simulink model "combined_experiment"  (R2020a)
settings: Solver=FixedStepAuto  StartTime=0.0  StopTime=tsim  FixedStep=baseRate  RelTol=1e-3  EnableMultiTasking=on
values from neighbouring files (symbols this model uses):
  a1 = str2double(environment_file(search_start(1)+length(value)+1:search_start(1)+search_end(1)-2))    [Run_Initializer.m]
  a2 = str2double(environment_file(search_start(1)+length(value)+1:search_start(1)+search_end(1)-2))    [Run_Initializer.m]
  a3 = str2double(environment_file(search_start(1)+length(value)+1:search_start(1)+search_end(1)-2))    [Run_Initializer.m]
  b0 = str2double(environment_file(search_start(1)+length(value)+1:search_start(1)+search_end(1)-2))    [Run_Initializer.m]
  b1 = str2double(environment_file(search_start(1)+length(value)+1:search_start(1)+search_end(1)-2))    [Run_Initializer.m]
  b2 = str2double(environment_file(search_start(1)+length(value)+1:search_start(1)+search_end(1)-2))    [Run_Initializer.m]
  baseRate = 1/20    (= 0.05)    [Run_Initializer.m]
  bring_arm_to_rest_time = 3    [Run_Initializer.m]
  drop_states_BLACK = [ 2.33; 1.2; target_starting_angle]    [Run_Initializer.m]
  drop_states_BLUE = [ xLength/2+0.9; yLength/2+0.5; 0]    [Run_Initializer.m]
  drop_states_RED = [ 0.5; 1.6; pi/4]    [Run_Initializer.m]
  elbow_max_omega = shoulder_max_omega    [Run_Initializer.m]
  F_red_X_nominal = 0.2196    [Run_Initializer.m]
  F_red_Y_nominal = 0.2825    [Run_Initializer.m]
  F_thrusters_BLACK = 0.183.*ones(8,1)    [Run_Initializer.m]
  F_thrusters_BLUE = 0.183.*ones(8,1)    [Run_Initializer.m]
  F_thrusters_RED = [F_red_X_nominal; F_red_X_nominal; F_red_Y_nominal; F_red_Y_nominal; F_red_X_nominal; F_red_X_nominal; F_red_Y_nominal; F_red_Y_nominal]    [Run_Initializer.m]
  home_states_BLACK = [ 2.33; 1.2; target_starting_angle]    [Run_Initializer.m]
  home_states_BLUE = [ xLength/2-0.9; yLength/2+0.5; 0]    [Run_Initializer.m]
  home_states_RED = drop_states_RED    [Run_Initializer.m]
  I0 = str2double(environment_file(search_start(1)+length(value)+1:search_start(1)+search_end(1)-2))    [Run_Initializer.m]
  I1 = str2double(environment_file(search_start(1)+length(value)+1:search_start(1)+search_end(1)-2))    [Run_Initializer.m]
  I2 = str2double(environment_file(search_start(1)+length(value)+1:search_start(1)+search_end(1)-2))    [Run_Initializer.m]
  I3 = str2double(environment_file(search_start(1)+length(value)+1:search_start(1)+search_end(1)-2))    [Run_Initializer.m]
  init_states_BLACK = [ 2.33; 1.2; target_starting_angle]    [Run_Initializer.m]
  init_states_BLUE = [ xLength/2+0.9; yLength/2+0.5; 0]    [Run_Initializer.m]
  init_states_RED = drop_states_RED    [Run_Initializer.m]
  joint_limit_buffer_angle = 0    [Run_Initializer.m]
  Kd_tb = 0.4/5    (= 0.08)    [Run_Initializer.m]
  Kd_tblue = 0.4    [Run_Initializer.m]
  Kd_tr = 0.4    [Run_Initializer.m]
  Kd_xb = 5    [Run_Initializer.m]
  Kd_xblue = 5    [Run_Initializer.m]
  Kd_xr = 5    [Run_Initializer.m]
  Kd_yb = 5    [Run_Initializer.m]
  Kd_yblue = 5    [Run_Initializer.m]
  Kd_yr = 5    [Run_Initializer.m]
  Kp_tb = 0.1/5    (= 0.02)    [Run_Initializer.m]
  Kp_tblue = 0.1    [Run_Initializer.m]
  Kp_tr = 0.1    [Run_Initializer.m]
  Kp_xb = 2    [Run_Initializer.m]
  Kp_xblue = 2    [Run_Initializer.m]
  Kp_xr = 2    [Run_Initializer.m]
  Kp_yb = 2    [Run_Initializer.m]
  Kp_yblue = 2    [Run_Initializer.m]
  Kp_yr = 2    [Run_Initializer.m]
  m0 = str2double(environment_file(search_start(1)+length(value)+1:search_start(1)+search_end(1)-2))    [Run_Initializer.m]
  m1 = str2double(environment_file(search_start(1)+length(value)+1:search_start(1)+search_end(1)-2))    [Run_Initializer.m]
  m2 = str2double(environment_file(search_start(1)+length(value)+1:search_start(1)+search_end(1)-2))    [Run_Initializer.m]
  m3 = str2double(environment_file(search_start(1)+length(value)+1:search_start(1)+search_end(1)-2))    [Run_Initializer.m]
  max_body_omega = str2num(erase(environment_file(search_start(1)+length(value)+1:search_start(1)+search_end(1)-2),'np.'))    [Run_Initializer.m]
  max_x_velocity = str2double(environment_file(search_start(1)+length(value)+1:search_start(1)+search_end(1)-2))    [Run_Initializer.m]
  max_y_velocity = max_x_velocity    [Run_Initializer.m]
  noise_variance_BLACK = 0    [Run_Initializer.m]
  noise_variance_BLUE = 0    [Run_Initializer.m]
  noise_variance_RED = 0    [Run_Initializer.m]
  Phase0_End = Phase0_Duration    (= 5)    [Run_Initializer.m]
  Phase1_End = Phase0_Duration + Phase1_Duration    (= 10)    [Run_Initializer.m]
  Phase2_End = Phase0_Duration + Phase1_Duration +                                   Phase2_Duration    (= 25)    [Run_Initializer.m]
  Phase3_End = Phase0_Duration + Phase1_Duration +                                   Phase2_Duration + Phase3_Duration    (= 205)    [Run_Initializer.m]
  Phase3_SubPhase1_End = Phase2_End + Phase3_SubPhase1_Duration    (= 55)    [Run_Initializer.m]
  Phase3_SubPhase2_End = Phase2_End + Phase3_SubPhase1_Duration +                                   Phase3_SubPhase2_Duration    (= 85)    [Run_Initializer.m]
  Phase3_SubPhase3_End = Phase2_End + Phase3_SubPhase1_Duration +                                   Phase3_SubPhase2_Duration +                                  Phase3_SubPhase3_Duration    (= 205)    [Run_Initializer.m]
  Phase3_SubPhase4_End = Phase2_End + Phase3_SubPhase1_Duration +                                   Phase3_SubPhase2_Duration +                                  Phase3_SubPhase3_Duration +                                  Phase3_SubPhase4_Duration    [Run_Initializer.m]
  Phase4_End = Phase0_Duration + Phase1_Duration +                                   Phase2_Duration + Phase3_Duration +                                   Phase4_Duration    (= 225)    [Run_Initializer.m]
  Phase5_End = Phase0_Duration + Phase1_Duration +                                   Phase2_Duration + Phase3_Duration +                                   Phase4_Duration + Phase5_Duration    (= 230)    [Run_Initializer.m]
  phi = str2num(erase(environment_file(search_start(1)+length(value)+1:search_start(1)+search_end(1)-2),'np.'))    [Run_Initializer.m]
  serverRate = 1/10    (= 0.1)    [Run_Initializer.m]
  shoulder_max_omega = str2num(erase(environment_file(search_start(1)+length(value)+1:search_start(1)+search_end(1)-2),'np.'))    [Run_Initializer.m]
  target_angular_velocity = -5*pi/180    (= -0.0872664625997)    [Run_Initializer.m]
  thruster_dist2CG_BLACK = [72.80;-65.20;61.75;-79.75;65.20;-65.20;74.25;-54.75]    [Run_Initializer.m]
  thruster_dist2CG_BLUE = [83.42;-52.58;55.94;-60.05;54.08;-53.92;77.06;-55.94]    [Run_Initializer.m]
  thruster_dist2CG_RED = [69.38;-56.62;50.01;-81.49;61.12;-68.38;78.99;-52.01]    [Run_Initializer.m]
  wrist_max_omega = shoulder_max_omega    [Run_Initializer.m]
undefined symbols (not defined in the file or in its folder): DiscIntNeverNeededParam, KI_vel_PI, KI_vel_PI_theta, Kp_vel_PI, Kp_vel_PI_theta, platformSelection, simMode, WhoAmI
libraries: dspstat3 x18, dspsigops x12, embdlinuxlib x10, raspberrypiBasiclib x10, MainLibrary x9, simulink x8, mspfiltlib x3, dsparch4 x3, dspswit3 x2, sensehatlib x1
(part 6 of 13)

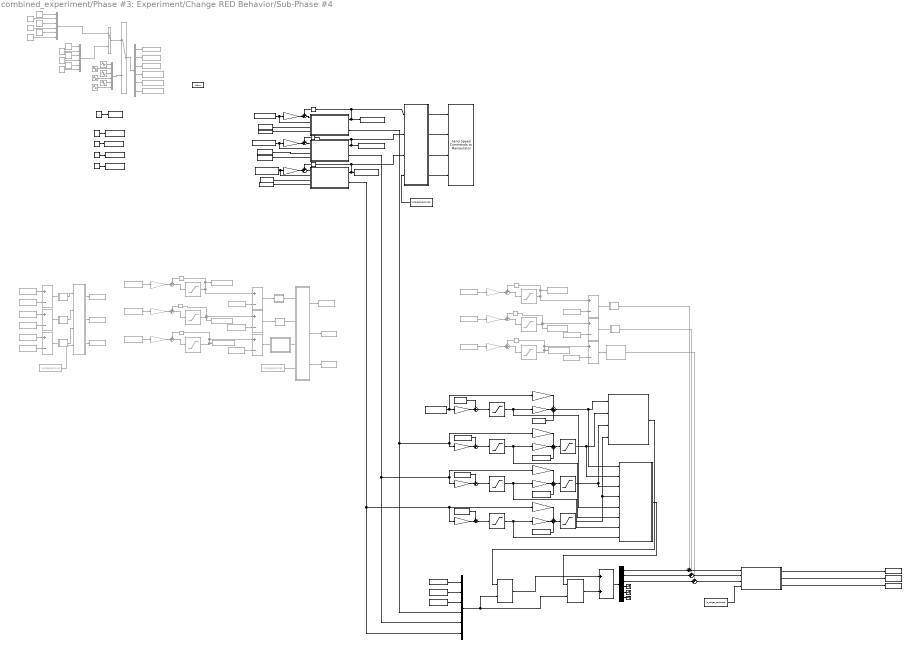
== system combined_experiment/Phase #3: Experiment/Change RED Behavior/Sub-Phase #4 ==
  note: desired q0
  note: desired q0_dot
      | (saturated)
  note: ARM Control Law - RED
  note: Acceleration-integral control law
  note: Additional Blocks
  note: Additional blocks are stored above. Note that to control attitude using the RW, simply replace RED_Tz with RED_Tz_RW.
  note: A simple PD control law is used here to command the platform to it's initial position, as defined in the initializer.
  note: This section is reserved for any control law for the robotic manipulator.
  note: Integrate and saturate acceleration signals to get desired velocities
  note: Velocity-PI control law
  note: Actually control it here
  note: Feedforward control
  note: desired q1_dot
      | (saturated)
  note: desired q1
  note: desired q2_dot
      | (saturated)
  note: desired q2
  note: desired q3_dot
      | (saturated)
  note: desired q3
  note: Velocity-PI control law
  note: Actually control it here
  note: OPTIONAL ADDITIONAL FEEDBACK VELOCITY PROPORTIONAL CONTROL
  Action Port : ActionPort  ActionPortLabel=elseif( u1 < u5)
  Check limits : MATLAB Function  TreatAsAtomicUnit=on
  Check limits1 : MATLAB Function  TreatAsAtomicUnit=on
  Check limits2 : MATLAB Function  TreatAsAtomicUnit=on
  Constant : Constant  Commented=on  Value=0.01
  Constant{1,4..6} (4 alike) : Constant  Value=0
  Constant2 : Constant  Commented=on  Value=-0.005
  Constant3 : Constant  Commented=on  Value=0.015
  Constant7 : Constant  Commented=on  Value=0.01
  Constant8 : Constant  Commented=on  Value=-0.01
  Constant9 : Constant  Commented=on  Value=0.01
  Custom Integral Acceleration Controller : Subsystem  Commented=on
  Custom Integral Acceleration Controller1 : Subsystem  Commented=on
  Custom Integral Acceleration Controller2 : Subsystem  Commented=on
  Data Store Read : DataStoreRead  DataStoreName=RED_Desired_alpha1
  Data Store Read1 : DataStoreRead  DataStoreName=RED_Desired_alpha2
  Data Store Read10 : DataStoreRead  DataStoreName=RED_omega3
  Data Store Read11 : DataStoreRead  DataStoreName=RED_omega2
  Data Store Read12 : DataStoreRead  DataStoreName=RED_omega1
  Data Store Read13 : DataStoreRead  DataStoreName=RED_theta3
  Data Store Read14 : DataStoreRead  DataStoreName=RED_theta2
  Data Store Read15 : DataStoreRead  DataStoreName=RED_theta1
  Data Store Read17 : DataStoreRead  Commented=on  DataStoreName=RED_Vx
  Data Store Read18 : DataStoreRead  Commented=on  DataStoreName=RED_Vy
  Data Store Read19 : DataStoreRead  DataStoreName=RED_theta1
  Data Store Read2 : DataStoreRead  DataStoreName=RED_Desired_alpha3
  Data Store Read20 : DataStoreRead  DataStoreName=RED_theta2
  Data Store Read21 : DataStoreRead  DataStoreName=RED_theta3
  Data Store Read22 : DataStoreRead  DataStoreName=RED_omega1
  Data Store Read23 : DataStoreRead  DataStoreName=RED_omega2
  Data Store Read24 : DataStoreRead  DataStoreName=RED_omega3
  Data Store Read25 : DataStoreRead  Commented=on  DataStoreName=RED_RzD
  Data Store Read26 : DataStoreRead  DataStoreName=RED_RzD
  Data Store Read27 : DataStoreRead  DataStoreName=RED_Rz
  Data Store Read3 : DataStoreRead  Commented=on  DataStoreName=is_target_captured
  Data Store Read4 : DataStoreRead  DataStoreName=is_target_captured
  Data Store Read5 : DataStoreRead  Commented=on  DataStoreName=is_target_captured
  Data Store Read6 : DataStoreRead  Commented=on  DataStoreName=RED_Vx
  Data Store Read7 : DataStoreRead  Commented=on  DataStoreName=RED_Vy
  Data Store Read8 : DataStoreRead  Commented=on  DataStoreName=RED_RzD
  Data Store Read9 : DataStoreRead  DataStoreName=is_target_captured
  Data Store Write : DataStoreWrite  DataStoreName=RED_Tz_Shoulder
  Data Store Write1 : DataStoreWrite  DataStoreName=RED_Tz_Elbow
  Data Store Write10 : DataStoreWrite  DataStoreName=RED_omega1_command
  Data Store Write11 : DataStoreWrite  DataStoreName=RED_omega2_command
  Data Store Write12 : DataStoreWrite  DataStoreName=RED_omega3_command
  Data Store Write13 : DataStoreWrite  Commented=on  DataStoreName=RED_Desired_Ax
  Data Store Write14 : DataStoreWrite  Commented=on  DataStoreName=RED_Desired_Ay
  Data Store Write15 : DataStoreWrite  Commented=on  DataStoreName=RED_Desired_Alpha
  Data Store Write16 : DataStoreWrite  Commented=on  DataStoreName=RED_Vy_command
  Data Store Write17 : DataStoreWrite  Commented=on  DataStoreName=RED_RzD_command
  Data Store Write18 : DataStoreWrite  Commented=on  DataStoreName=RED_Vx_command
  Data Store Write19 : DataStoreWrite  Commented=on  DataStoreName=RED_Desired_alpha1
  Data Store Write2 : DataStoreWrite  DataStoreName=RED_Tz_Wrist
  Data Store Write20 : DataStoreWrite  Commented=on  DataStoreName=RED_Desired_alpha2
  Data Store Write21 : DataStoreWrite  Commented=on  DataStoreName=RED_Desired_alpha3
  Data Store Write22 : DataStoreWrite  Commented=on  DataStoreName=RED_Vy_command
  Data Store Write23 : DataStoreWrite  Commented=on  DataStoreName=RED_RzD_command
  Data Store Write24 : DataStoreWrite  Commented=on  DataStoreName=RED_Vx_command
  Data Store Write3 : DataStoreWrite  DataStoreName=Float_State
  Delay{1..2,6..9} (6 alike) : Delay  Commented=on  DelayLength=1
  Delay3 : Delay  DelayLength=1
  Delay4 : Delay  DelayLength=1
  Delay5 : Delay  DelayLength=1
  Demux : Demux  Commented=on  Outputs=6
  Demux1 : Demux  Outputs=6
  Gain{,1..2,6,8..9,11,13..14,16..17} (11 alike) : Gain  Gain=serverRate
  Gain{7,10,12,15} (4 alike) : Gain  Gain=0.5*serverRate^2
  Gain{3..5,18..20} (6 alike) : Gain  Commented=on  Gain=serverRate
  Manual Switch : ManualSwitch  Commented=on
  Manual Switch1 : ManualSwitch  Commented=on
  Mux : Mux  Commented=on  Inputs=6
  Mux1 : Mux  Commented=on  Inputs=6
  Mux2 : Mux  Commented=on  Inputs=6
  Mux3 : Mux  Inputs=6
  PI Velocity Controller Theta : Subsystem  Commented=on
  PI Velocity Controller Theta1 : Subsystem  Commented=on
  PI Velocity Controller X : Subsystem  Commented=on
  PI Velocity Controller X1 : Subsystem  Commented=on
  PI Velocity Controller X2 : Subsystem  Commented=on
  PI Velocity Controller X3 : Subsystem  Commented=on
  Product : Product  Multiplication=Matrix(*)
  Product1 : Product  Multiplication=Matrix(*)
  Puck State : Constant
  RED_Fx1 : DataStoreWrite  Commented=on  DataStoreName=RED_Fx
  RED_Fx2 : DataStoreWrite  Commented=on  DataStoreName=RED_Fx
  RED_Fx3 : DataStoreWrite  DataStoreName=RED_Fx
  RED_Fy1 : DataStoreWrite  Commented=on  DataStoreName=RED_Fy
  RED_Fy2 : DataStoreWrite  Commented=on  DataStoreName=RED_Fy
  RED_Fy3 : DataStoreWrite  DataStoreName=RED_Fy
  RED_Py 1 : DataStoreRead  Commented=on  DataStoreName=RED_Desired_Ay
  RED_Py 10 : DataStoreRead  DataStoreName=RED_Desired_Ax
  RED_Py 2 : DataStoreRead  Commented=on  DataStoreName=RED_Desired_Ay
  RED_Py 3 : DataStoreRead  Commented=on  DataStoreName=RED_Desired_Ax
  RED_Py 4 : DataStoreRead  Commented=on  DataStoreName=RED_Desired_Ax
  RED_Py 5 : DataStoreRead  Commented=on  DataStoreName=RED_Ay
  RED_Py 6 : DataStoreRead  Commented=on  DataStoreName=RED_Desired_Ay
  RED_Py 7 : DataStoreRead  Commented=on  DataStoreName=RED_Desired_Ax
  RED_Py 8 : DataStoreRead  Commented=on  DataStoreName=RED_Ax
  RED_Py 9 : DataStoreRead  DataStoreName=RED_Desired_Ay
  RED_Rz1 : DataStoreRead  Commented=on  DataStoreName=RED_Desired_Alpha
  RED_Rz2 : DataStoreRead  Commented=on  DataStoreName=RED_Desired_Alpha
  RED_Rz3 : DataStoreRead  Commented=on  DataStoreName=RED_Desired_Alpha
  RED_Rz4 : DataStoreRead  Commented=on  DataStoreName=RED_RzDD
  RED_Rz5 : DataStoreRead  DataStoreName=RED_Desired_Alpha
  RED_Rz6 : DataStoreRead  DataStoreName=RED_Desired_Alpha
  RED_Tz1 : DataStoreWrite  Commented=on  DataStoreName=RED_Tz
  RED_Tz2 : DataStoreWrite  DataStoreName=RED_Tz
  RED_Tz3 : DataStoreWrite  Commented=on  DataStoreName=RED_Tz
  RED_Tz_RW : DataStoreWrite  DataStoreName=RED_Tz_RW
  Saturage body angular velocity command1 : Saturate  UpperLimit=shoulder_max_omega  LowerLimit=-shoulder_max_omega
  Saturage body angular velocity command2 : Saturate  UpperLimit=max_body_omega  LowerLimit=-max_body_omega
  Saturage body angular velocity command3 : Saturate  UpperLimit=elbow_max_omega  LowerLimit=-elbow_max_omega
  Saturage body angular velocity command4 : Saturate  UpperLimit=wrist_max_omega  LowerLimit=-wrist_max_omega
  Saturage body angular velocity command : Saturate  Commented=on  UpperLimit=max_body_omega  LowerLimit=-max_body_omega
  Saturage body angular velocity command1 : Saturate  Commented=on  UpperLimit=max_body_omega  LowerLimit=-max_body_omega
  Saturate velocity command X : Saturate  Commented=on  UpperLimit=max_x_velocity  LowerLimit=-max_x_velocity
  Saturate velocity command X1 : Saturate  Commented=on  UpperLimit=max_x_velocity  LowerLimit=-max_x_velocity
  Saturate velocity command Y : Saturate  Commented=on  UpperLimit=max_y_velocity  LowerLimit=-max_y_velocity
  Saturate velocity command Y1 : Saturate  Commented=on  UpperLimit=max_y_velocity  LowerLimit=-max_y_velocity
  Send Speed Commands to Manipulator : MainLibrary/Dynamixel Functions/Send Speed Commands to  Manipulator
      settings: SourceProductName=SPOT Custom Library
  Sine Wave : Sin  Commented=on  Amplitude=0.015
  Sine Wave1 : Sin  Commented=on  Amplitude=0.015  Phase=pi
  Sine Wave2 : Sin  Commented=on  Amplitude=0.04
  Sine Wave3 : Sin  Commented=on  Amplitude=0.015
  Sine Wave4 : Sin  Commented=on  Amplitude=0.015  Phase=pi
  Sine Wave5 : Sin  Commented=on  Amplitude=0.04
  Subtract{1..9} (9 alike) : Sum  Commented=on  Inputs=+-
  Sum : Sum
  Sum{1..2,6,15..17} (6 alike) : Sum  Commented=on  Inputs=++|
  Sum{3..5,8,10,12..13,18..20} (10 alike) : Sum  Inputs=++|
  Sum{7,9,11,14} (4 alike) : Sum  Inputs=+++
  Terminator : Terminator
  Terminator1 : Terminator
  Terminator2 : Terminator
  Uniform Random Number{,1,3..4} (4 alike) : UniformRandomNumber  Commented=on  Minimum=-0.015  Maximum=0.015
  Uniform Random Number2 : UniformRandomNumber  Commented=on  Minimum=-0.04  Maximum=0.04
  Uniform Random Number5 : UniformRandomNumber  Commented=on  Minimum=-0.04  Maximum=0.04
  calculate_coriolis_matrix : MATLAB Function  TreatAsAtomicUnit=on
  calculate_mass_matrix : MATLAB Function  TreatAsAtomicUnit=on
  saturate arm angle : Saturate  UpperLimit=pi/2  LowerLimit=-pi/2
  saturate arm angle1 : Saturate  UpperLimit=pi/2  LowerLimit=-pi/2
  saturate arm angle2 : Saturate  UpperLimit=pi/2  LowerLimit=-pi/2
  wind down upon capture : MATLAB Function  TreatAsAtomicUnit=on
  wind down upon_capture : MATLAB Function  Commented=on  TreatAsAtomicUnit=on
  wind down upon_capture1 : MATLAB Function  Commented=on  TreatAsAtomicUnit=on
  wind down upon_capture2 : MATLAB Function  TreatAsAtomicUnit=on
  wires:
  Constant1/1 -> RED_Tz_RW/1
  Constant6/1 -> Data Store Write2/1
  Constant4/1 -> Data Store Write/1
  Constant5/1 -> Data Store Write1/1
  Puck State/1 -> Data Store Write3/1
  Subtract6/1 -> Custom Integral Acceleration Controller1/1(ey)
  Subtract5/1 -> Custom Integral Acceleration Controller/1(ex)
  RED_Py 8/1 -> Subtract5/2
  RED_Rz4/1 -> Subtract7/2
  Subtract7/1 -> Custom Integral Acceleration Controller2/1(ez)
  RED_Py 5/1 -> Subtract6/2
  RED_Py 3/1 -> Subtract5/1
  RED_Py 1/1 -> Subtract6/1
  RED_Rz1/1 -> Subtract7/1
  Data Store Read/1 -> Check limits/2(alpha_command), Gain/1
  Check limits/1(saturated_omega) -> wind down upon capture/1(omega1_in), Delay3/1, Data Store Write10/1
  Delay3/1 -> Sum3/1
  Gain/1 -> Sum3/2
  Sum3/1 -> Check limits/1(omega_command)
  Sum4/1 -> Check limits1/1(omega_command)
  Delay4/1 -> Sum4/1
  Gain1/1 -> Sum4/2
  Check limits1/1(saturated_omega) -> Data Store Write11/1, wind down upon capture/2(omega2_in), Delay4/1
  Sum5/1 -> Check limits2/1(omega_command)
  Delay5/1 -> Sum5/1
  Gain2/1 -> Sum5/2
  Check limits2/1(saturated_omega) -> Data Store Write12/1, wind down upon capture/3(omega3_in), Delay5/1
  Data Store Read2/1 -> Check limits2/2(alpha_command), Gain2/1
  Data Store Read1/1 -> Check limits1/2(alpha_command), Gain1/1
  Data Store Read3/1 -> wind down upon_capture/4(is_target_captured)
  Custom Integral Acceleration Controller/1(Fx) -> wind down upon_capture/1(Fx_in)
  Custom Integral Acceleration Controller1/1(Fy) -> wind down upon_capture/2(Fy_in)
  Custom Integral Acceleration Controller2/1(Tz) -> wind down upon_capture/3(Tz_in)
  wind down upon capture/4(accel_time_ms) -> Send Speed Commands to Manipulator/4
  wind down upon_capture/1(Fx_out) -> RED_Fx2/1
  wind down upon_capture/2(Fy_out) -> RED_Fy2/1
  wind down upon_capture/3(Tz_out) -> RED_Tz3/1
  Sine Wave/1 -> Mux/1
  Mux/1 -> Manual Switch/2
  Constant3/1 -> Mux1/3
  Constant2/1 -> Mux1/2
  Constant/1 -> Mux1/1
  Manual Switch/1 -> Demux/1
  Demux/1 -> Data Store Write13/1
  Demux/2 -> Data Store Write14/1
  Demux/3 -> Data Store Write15/1
  Data Store Read4/1 -> wind down upon capture/4(is_target_captured)
  Subtract2/1 -> PI Velocity Controller X1/1(e_Vx)
  PI Velocity Controller X1/1(Fx) -> wind down upon_capture1/2(Fy_in)
  wind down upon_capture1/3(Tz_out) -> RED_Tz1/1
  PI Velocity Controller Theta/1(F_omega) -> wind down upon_capture1/3(Tz_in)
  Data Store Read5/1 -> wind down upon_capture1/4(is_target_captured)
  PI Velocity Controller X/1(Fx) -> wind down upon_capture1/1(Fx_in)
  wind down upon_capture1/1(Fx_out) -> RED_Fx1/1
  Subtract1/1 -> PI Velocity Controller X/1(e_Vx)
  Subtract3/1 -> PI Velocity Controller Theta/1(e_omega)
  wind down upon_capture1/2(Fy_out) -> RED_Fy1/1
  Sum2/1 -> Saturate velocity command Y/1
  Saturate velocity command Y/1 -> Data Store Write16/1, Delay2/1, Subtract2/1
  Gain4/1 -> Sum2/2
  Gain5/1 -> Sum6/2
  Sum6/1 -> Saturage body angular velocity command/1
  Delay1/1 -> Sum1/1
  RED_Py 2/1 -> Gain4/1
  Delay6/1 -> Sum6/1
  Delay2/1 -> Sum2/1
  Gain3/1 -> Sum1/2
  Saturage body angular velocity command/1 -> Subtract3/1, Delay6/1, Data Store Write17/1
  RED_Rz2/1 -> Gain5/1
  Sum1/1 -> Saturate velocity command X/1
  RED_Py 4/1 -> Gain3/1
  Saturate velocity command X/1 -> Delay1/1, Data Store Write18/1, Subtract1/1
  Data Store Read6/1 -> Subtract1/2
  Data Store Read7/1 -> Subtract2/2
  Data Store Read8/1 -> Subtract3/2
  Manual Switch1/1 -> Manual Switch/1
  Mux1/1 -> Manual Switch1/1
  Uniform Random Number/1 -> Mux2/1
  Mux2/1 -> Manual Switch1/2
  Uniform Random Number2/1 -> Mux2/3
  Uniform Random Number1/1 -> Mux2/2
  RED_Py 10/1 -> Mux3/1
  RED_Py 9/1 -> Mux3/2
  RED_Rz5/1 -> Mux3/3
  Check limits/2(saturated_alpha) -> Mux3/4, Gain8/1, Gain10/1
  Check limits1/2(saturated_alpha) -> Gain13/1, Gain12/1, Mux3/5
  Check limits2/2(saturated_alpha) -> Gain16/1, Gain15/1, Mux3/6
  Mux3/1 -> Product1/2, Product/2
  calculate_mass_matrix/1(M) -> Product/1
  calculate_coriolis_matrix/1(C) -> Product1/1
  Product1/1 -> Sum/2
  Product/1 -> Sum/1
  Sum/1 -> Demux1/1
  Data Store Read9/1 -> wind down upon_capture2/4(is_target_captured)
  Demux1/4 -> Terminator/1
  Demux1/6 -> Terminator2/1
  Demux1/5 -> Terminator1/1
  Gain11/1 -> Sum12/2
  RED_Rz6/1 -> Gain7/1, Gain11/1
  Sum12/1 -> Saturage body angular velocity command2/1
  Data Store Read26/1 -> Sum12/1
  Saturage body angular velocity command2/1 -> calculate_coriolis_matrix/5(q0_dot_d), Gain6/1
  Gain6/1 -> Sum7/2
  Gain7/1 -> Sum7/1
  Data Store Read27/1 -> Sum7/3
  Sum7/1 -> calculate_coriolis_matrix/1(q0_d), calculate_mass_matrix/1(q0_d)
  Data Store Read22/1 -> Sum8/1
  Sum8/1 -> Saturage body angular velocity command1/1
  Gain8/1 -> Sum8/2
  Gain10/1 -> Sum9/1
  Sum9/1 -> saturate arm angle/1
  Data Store Read19/1 -> Sum9/3
  Gain9/1 -> Sum9/2
  Saturage body angular velocity command1/1 -> calculate_coriolis_matrix/6(q1_dot_d), Gain9/1
  Data Store Read20/1 -> Sum11/3
  Gain13/1 -> Sum10/2
  Sum10/1 -> Saturage body angular velocity command3/1
  Saturage body angular velocity command3/1 -> calculate_coriolis_matrix/7(q2_dot_d), Gain14/1
  Sum11/1 -> saturate arm angle1/1
  Data Store Read23/1 -> Sum10/1
  Gain14/1 -> Sum11/2
  Gain12/1 -> Sum11/1
  Data Store Read21/1 -> Sum14/3
  Gain16/1 -> Sum13/2
  Sum13/1 -> Saturage body angular velocity command4/1
  Saturage body angular velocity command4/1 -> calculate_coriolis_matrix/8(q3_dot_d), Gain17/1
  Sum14/1 -> saturate arm angle2/1
  Data Store Read24/1 -> Sum13/1
  Gain17/1 -> Sum14/2
  Gain15/1 -> Sum14/1
  saturate arm angle/1 -> calculate_mass_matrix/2(q1_d), calculate_coriolis_matrix/2(q1_d)
  saturate arm angle1/1 -> calculate_coriolis_matrix/3(q2_d), calculate_mass_matrix/3(q2_d)
  saturate arm angle2/1 -> calculate_mass_matrix/4(q3_d), calculate_coriolis_matrix/4(q3_d)
  Demux/4 -> Data Store Write19/1
  Demux/5 -> Data Store Write20/1
  Demux/6 -> Data Store Write21/1
  Constant8/1 -> Mux1/5
  Constant7/1 -> Mux1/4
  Constant9/1 -> Mux1/6
  Sine Wave1/1 -> Mux/2
  Sine Wave2/1 -> Mux/3
  Uniform Random Number4/1 -> Mux2/5
  Uniform Random Number3/1 -> Mux2/4
  Uniform Random Number5/1 -> Mux2/6
  Sine Wave4/1 -> Mux/5
  Sine Wave3/1 -> Mux/4
  Sine Wave5/1 -> Mux/6
  Delay8/1 -> Sum16/1
  Delay7/1 -> Sum15/1
  Delay9/1 -> Sum17/1
  Sum15/1 -> Saturate velocity command X1/1
  RED_Py 7/1 -> Gain18/1
  RED_Py 6/1 -> Gain19/1
  Gain18/1 -> Sum15/2
  Saturate velocity command X1/1 -> Delay7/1, Data Store Write24/1, Subtract4/1
  Gain20/1 -> Sum17/2
  Gain19/1 -> Sum16/2
  Saturate velocity command Y1/1 -> Data Store Write22/1, Delay8/1, Subtract8/1
  RED_Rz3/1 -> Gain20/1
  Sum16/1 -> Saturate velocity command Y1/1
  Saturage body angular velocity command1/1 -> Subtract9/1, Delay9/1, Data Store Write23/1
  Subtract9/1 -> PI Velocity Controller Theta1/1(e_omega)
  Subtract4/1 -> PI Velocity Controller X2/1(e_Vx)
  Data Store Read17/1 -> Subtract4/2
  PI Velocity Controller X3/1(Fx) -> Sum19/1
  Data Store Read25/1 -> Subtract9/2
  Subtract8/1 -> PI Velocity Controller X3/1(e_Vx)
  PI Velocity Controller X2/1(Fx) -> Sum18/1
  Sum17/1 -> Saturage body angular velocity command1/1
  PI Velocity Controller Theta1/1(F_omega) -> Sum20/1
  Data Store Read18/1 -> Subtract8/2
  Demux1/1 -> Sum18/2
  Sum18/1 -> wind down upon_capture2/1(Fx_in)
  Sum20/1 -> wind down upon_capture2/3(Tz_in)
  Demux1/3 -> Sum20/2
  Sum19/1 -> wind down upon_capture2/2(Fy_in)
  Demux1/2 -> Sum19/2
  wind down upon capture/2(omega2_out) -> Send Speed Commands to Manipulator/2
  wind down upon capture/1(omega1_out) -> Send Speed Commands to Manipulator/1
  wind down upon capture/3(omega3_out) -> Send Speed Commands to Manipulator/3
  Data Store Read12/1 -> Check limits/4(current_omega)
  Data Store Read15/1 -> Check limits/3(current_theta)
  Data Store Read14/1 -> Check limits1/3(current_theta)
  Data Store Read11/1 -> Check limits1/4(current_omega)
  Data Store Read13/1 -> Check limits2/3(current_theta)
  Data Store Read10/1 -> Check limits2/4(current_omega)
  wind down upon_capture2/1(Fx_out) -> RED_Fx3/1
  wind down upon_capture2/2(Fy_out) -> RED_Fy3/1
  wind down upon_capture2/3(Tz_out) -> RED_Tz2/1

== system combined_experiment/Phase #3: Experiment/Change RED Behavior/Subsystem ==
  Universal_Time : DataStoreRead  DataStoreName=Univ_Time
  Time : Outport  VectorParamsAs1DForOutWhenUnconnected=off
  wires:
  Universal_Time/1 -> Time/1

== system combined_experiment/Phase #4: Return Home/Change BLACK Behavior/Custom Discrete PD (Attitude) ==
  ez : Inport
  Sum3 : Sum
  kd_tb : Gain  Gain=Kd_tb
  kp_tb : Gain  Gain=Kp_tb
  "x_dot -> x1" : Subsystem
  Tz : Outport  VectorParamsAs1DForOutWhenUnconnected=off
  wires:
  kd_tb/1 -> Sum3/1
  Sum3/1 -> Tz/1
  kp_tb/1 -> Sum3/2
  "x_dot -> x1"/1(dy(t)/dt) -> kd_tb/1
  ez/1 -> "x_dot -> x1"/1(y(t)), kp_tb/1

== system combined_experiment/Phase #4: Return Home/Change BLACK Behavior/Custom Discrete PD (X-Position) ==
  ex : Inport
  Sum3 : Sum
  kd_xb : Gain  Gain=Kd_xb
  kp_xb : Gain  Gain=Kp_xb
  "x_dot -> x1" : Subsystem
  Fx : Outport  VectorParamsAs1DForOutWhenUnconnected=off
  wires:
  kd_xb/1 -> Sum3/1
  ex/1 -> "x_dot -> x1"/1(y(t)), kp_xb/1
  kp_xb/1 -> Sum3/2
  "x_dot -> x1"/1(dy(t)/dt) -> kd_xb/1
  Sum3/1 -> Fx/1

== system combined_experiment/Phase #4: Return Home/Change BLACK Behavior/Custom Discrete PD (Y-Position) ==
  ey : Inport
  Sum3 : Sum
  kd_yb : Gain  Gain=Kd_yb
  kp_yb : Gain  Gain=Kp_yb
  "x_dot -> x1" : Subsystem
  Fy : Outport  VectorParamsAs1DForOutWhenUnconnected=off
  wires:
  kd_yb/1 -> Sum3/1
  Sum3/1 -> Fy/1
  kp_yb/1 -> Sum3/2
  "x_dot -> x1"/1(dy(t)/dt) -> kd_yb/1
  ey/1 -> "x_dot -> x1"/1(y(t)), kp_yb/1

== system combined_experiment/Phase #4: Return Home/Change BLACK Behavior/Hough Control ==
  Ref : Inport
  Act : Inport  Port=2
  MATLAB Function2 : MATLAB Function  TreatAsAtomicUnit=on
  MATLAB Function3 : MATLAB Function  TreatAsAtomicUnit=on
  MATLAB Function4 : MATLAB Function  TreatAsAtomicUnit=on
  Subtract2 : Sum  Inputs=+-
  Err : Outport  VectorParamsAs1DForOutWhenUnconnected=off
  wires:
  MATLAB Function4/1(e_out) -> Err/1
  MATLAB Function2/1(Oy) -> MATLAB Function4/1(Oy)
  Subtract2/1 -> MATLAB Function4/2(e_in)
  MATLAB Function2/2(Ox) -> Subtract2/1
  Act/1 -> MATLAB Function3/1(z)
  Ref/1 -> MATLAB Function2/1(z)
  MATLAB Function3/1(Ox) -> Subtract2/2

== system combined_experiment/Phase #4: Return Home/Change BLUE Behavior/Custom Discrete PD (Attitude) ==
  ez : Inport
  Sum3 : Sum
  kd_tb : Gain  Gain=Kd_tblue
  kp_tb : Gain  Gain=Kp_tblue
  "x_dot -> x1" : Subsystem
  Tz : Outport  VectorParamsAs1DForOutWhenUnconnected=off
  wires:
  kd_tb/1 -> Sum3/1
  Sum3/1 -> Tz/1
  kp_tb/1 -> Sum3/2
  "x_dot -> x1"/1(dy(t)/dt) -> kd_tb/1
  ez/1 -> "x_dot -> x1"/1(y(t)), kp_tb/1

== system combined_experiment/Phase #4: Return Home/Change BLUE Behavior/Custom Discrete PD (X-Position) ==
  ex : Inport
  Sum3 : Sum
  kd_xb : Gain  Gain=Kd_xblue
  kp_xb : Gain  Gain=Kp_xblue
  "x_dot -> x1" : Subsystem
  Fx : Outport  VectorParamsAs1DForOutWhenUnconnected=off
  wires:
  kd_xb/1 -> Sum3/1
  ex/1 -> "x_dot -> x1"/1(y(t)), kp_xb/1
  kp_xb/1 -> Sum3/2
  "x_dot -> x1"/1(dy(t)/dt) -> kd_xb/1
  Sum3/1 -> Fx/1

== system combined_experiment/Phase #4: Return Home/Change BLUE Behavior/Custom Discrete PD (Y-Position) ==
  ey : Inport
  Sum3 : Sum
  kd_yb : Gain  Gain=Kd_yblue
  kp_yb : Gain  Gain=Kp_yblue
  "x_dot -> x1" : Subsystem
  Fy : Outport  VectorParamsAs1DForOutWhenUnconnected=off
  wires:
  kd_yb/1 -> Sum3/1
  Sum3/1 -> Fy/1
  kp_yb/1 -> Sum3/2
  "x_dot -> x1"/1(dy(t)/dt) -> kd_yb/1
  ey/1 -> "x_dot -> x1"/1(y(t)), kp_yb/1

== system combined_experiment/Phase #4: Return Home/Change BLUE Behavior/Hough Control ==
  Ref : Inport
  Act : Inport  Port=2
  MATLAB Function2 : MATLAB Function  TreatAsAtomicUnit=on
  MATLAB Function3 : MATLAB Function  TreatAsAtomicUnit=on
  MATLAB Function4 : MATLAB Function  TreatAsAtomicUnit=on
  Subtract2 : Sum  Inputs=+-
  Err : Outport  VectorParamsAs1DForOutWhenUnconnected=off
  wires:
  MATLAB Function4/1(e_out) -> Err/1
  MATLAB Function2/1(Oy) -> MATLAB Function4/1(Oy)
  Subtract2/1 -> MATLAB Function4/2(e_in)
  MATLAB Function2/2(Ox) -> Subtract2/1
  Act/1 -> MATLAB Function3/1(z)
  Ref/1 -> MATLAB Function2/1(z)
  MATLAB Function3/1(Ox) -> Subtract2/2

== system combined_experiment/Phase #4: Return Home/Change RED Behavior/Custom Discrete PD (Attitude) ==
  ez : Inport
  Sum3 : Sum
  kd_tr : Gain  Gain=Kd_tr
  kp_tr : Gain  Gain=Kp_tr
  "x_dot -> x1" : Subsystem
  Tz : Outport  VectorParamsAs1DForOutWhenUnconnected=off
  wires:
  kd_tr/1 -> Sum3/1
  Sum3/1 -> Tz/1
  kp_tr/1 -> Sum3/2
  "x_dot -> x1"/1(dy(t)/dt) -> kd_tr/1
  ez/1 -> "x_dot -> x1"/1(y(t)), kp_tr/1

== system combined_experiment/Phase #4: Return Home/Change RED Behavior/Custom Discrete PD (X-Position) ==
  ex : Inport
  Sum3 : Sum
  kd_xr : Gain  Gain=Kd_xr
  kp_xr : Gain  Gain=Kp_xr
  "x_dot -> x1" : Subsystem
  Fx : Outport  VectorParamsAs1DForOutWhenUnconnected=off
  wires:
  kd_xr/1 -> Sum3/1
  ex/1 -> "x_dot -> x1"/1(y(t)), kp_xr/1
  kp_xr/1 -> Sum3/2
  "x_dot -> x1"/1(dy(t)/dt) -> kd_xr/1
  Sum3/1 -> Fx/1

== system combined_experiment/Phase #4: Return Home/Change RED Behavior/Custom Discrete PD (Y-Position) ==
  ey : Inport
  Sum3 : Sum
  kd_yr : Gain  Gain=Kd_yr
  kp_yr : Gain  Gain=Kp_yr
  "x_dot -> x1" : Subsystem
  Fy : Outport  VectorParamsAs1DForOutWhenUnconnected=off
  wires:
  kd_yr/1 -> Sum3/1
  Sum3/1 -> Fy/1
  kp_yr/1 -> Sum3/2
  "x_dot -> x1"/1(dy(t)/dt) -> kd_yr/1
  ey/1 -> "x_dot -> x1"/1(y(t)), kp_yr/1

== system combined_experiment/Phase #4: Return Home/Change RED Behavior/Hough Control ==
  Ref : Inport
  Act : Inport  Port=2
  MATLAB Function2 : MATLAB Function  TreatAsAtomicUnit=on
  MATLAB Function3 : MATLAB Function  TreatAsAtomicUnit=on
  MATLAB Function4 : MATLAB Function  TreatAsAtomicUnit=on
  Subtract2 : Sum  Inputs=+-
  Err : Outport  VectorParamsAs1DForOutWhenUnconnected=off
  wires:
  MATLAB Function4/1(e_out) -> Err/1
  MATLAB Function2/1(Oy) -> MATLAB Function4/1(Oy)
  Subtract2/1 -> MATLAB Function4/2(e_in)
  MATLAB Function2/2(Ox) -> Subtract2/1
  Act/1 -> MATLAB Function3/1(z)
  Ref/1 -> MATLAB Function2/1(z)
  MATLAB Function3/1(Ox) -> Subtract2/2

== system combined_experiment/Phase #5: Hold Home/Change BLACK Behavior/Custom Discrete PD (Attitude) ==
  ez : Inport
  Sum3 : Sum
  kd_tb : Gain  Gain=Kd_tb
  kp_tb : Gain  Gain=Kp_tb
  "x_dot -> x1" : Subsystem
  Tz : Outport  VectorParamsAs1DForOutWhenUnconnected=off
  wires:
  kd_tb/1 -> Sum3/1
  Sum3/1 -> Tz/1
  kp_tb/1 -> Sum3/2
  "x_dot -> x1"/1(dy(t)/dt) -> kd_tb/1
  ez/1 -> "x_dot -> x1"/1(y(t)), kp_tb/1

== system combined_experiment/Phase #5: Hold Home/Change BLACK Behavior/Custom Discrete PD (X-Position) ==
  ex : Inport
  Sum3 : Sum
  kd_xb : Gain  Gain=Kd_xb
  kp_xb : Gain  Gain=Kp_xb
  "x_dot -> x1" : Subsystem
  Fx : Outport  VectorParamsAs1DForOutWhenUnconnected=off
  wires:
  kd_xb/1 -> Sum3/1
  ex/1 -> "x_dot -> x1"/1(y(t)), kp_xb/1
  kp_xb/1 -> Sum3/2
  "x_dot -> x1"/1(dy(t)/dt) -> kd_xb/1
  Sum3/1 -> Fx/1

== system combined_experiment/Phase #5: Hold Home/Change BLACK Behavior/Custom Discrete PD (Y-Position) ==
  ey : Inport
  Sum3 : Sum
  kd_yb : Gain  Gain=Kd_yb
  kp_yb : Gain  Gain=Kp_yb
  "x_dot -> x1" : Subsystem
  Fy : Outport  VectorParamsAs1DForOutWhenUnconnected=off
  wires:
  kd_yb/1 -> Sum3/1
  Sum3/1 -> Fy/1
  kp_yb/1 -> Sum3/2
  "x_dot -> x1"/1(dy(t)/dt) -> kd_yb/1
  ey/1 -> "x_dot -> x1"/1(y(t)), kp_yb/1

== system combined_experiment/Phase #5: Hold Home/Change BLACK Behavior/Hough Control ==
  Ref : Inport
  Act : Inport  Port=2
  MATLAB Function2 : MATLAB Function  TreatAsAtomicUnit=on
  MATLAB Function3 : MATLAB Function  TreatAsAtomicUnit=on
  MATLAB Function4 : MATLAB Function  TreatAsAtomicUnit=on
  Subtract2 : Sum  Inputs=+-
  Err : Outport  VectorParamsAs1DForOutWhenUnconnected=off
  wires:
  MATLAB Function4/1(e_out) -> Err/1
  MATLAB Function2/1(Oy) -> MATLAB Function4/1(Oy)
  Subtract2/1 -> MATLAB Function4/2(e_in)
  MATLAB Function2/2(Ox) -> Subtract2/1
  Act/1 -> MATLAB Function3/1(z)
  Ref/1 -> MATLAB Function2/1(z)
  MATLAB Function3/1(Ox) -> Subtract2/2

== system combined_experiment/Phase #5: Hold Home/Change BLUE Behavior/Custom Discrete PD (Attitude) ==
  ez : Inport
  Sum3 : Sum
  kd_tb : Gain  Gain=Kd_tblue
  kp_tb : Gain  Gain=Kp_tblue
  "x_dot -> x1" : Subsystem
  Tz : Outport  VectorParamsAs1DForOutWhenUnconnected=off
  wires:
  kd_tb/1 -> Sum3/1
  Sum3/1 -> Tz/1
  kp_tb/1 -> Sum3/2
  "x_dot -> x1"/1(dy(t)/dt) -> kd_tb/1
  ez/1 -> "x_dot -> x1"/1(y(t)), kp_tb/1

== system combined_experiment/Phase #5: Hold Home/Change BLUE Behavior/Custom Discrete PD (X-Position) ==
  ex : Inport
  Sum3 : Sum
  kd_xb : Gain  Gain=Kd_xblue
  kp_xb : Gain  Gain=Kp_xblue
  "x_dot -> x1" : Subsystem
  Fx : Outport  VectorParamsAs1DForOutWhenUnconnected=off
  wires:
  kd_xb/1 -> Sum3/1
  ex/1 -> "x_dot -> x1"/1(y(t)), kp_xb/1
  kp_xb/1 -> Sum3/2
  "x_dot -> x1"/1(dy(t)/dt) -> kd_xb/1
  Sum3/1 -> Fx/1

== system combined_experiment/Phase #5: Hold Home/Change BLUE Behavior/Custom Discrete PD (Y-Position) ==
  ey : Inport
  Sum3 : Sum
  kd_yb : Gain  Gain=Kd_yblue
  kp_yb : Gain  Gain=Kp_yblue
  "x_dot -> x1" : Subsystem
  Fy : Outport  VectorParamsAs1DForOutWhenUnconnected=off
  wires:
  kd_yb/1 -> Sum3/1
  Sum3/1 -> Fy/1
  kp_yb/1 -> Sum3/2
  "x_dot -> x1"/1(dy(t)/dt) -> kd_yb/1
  ey/1 -> "x_dot -> x1"/1(y(t)), kp_yb/1

== system combined_experiment/Phase #5: Hold Home/Change BLUE Behavior/Hough Control ==
  Ref : Inport
  Act : Inport  Port=2
  MATLAB Function2 : MATLAB Function  TreatAsAtomicUnit=on
  MATLAB Function3 : MATLAB Function  TreatAsAtomicUnit=on
  MATLAB Function4 : MATLAB Function  TreatAsAtomicUnit=on
  Subtract2 : Sum  Inputs=+-
  Err : Outport  VectorParamsAs1DForOutWhenUnconnected=off
  wires:
  MATLAB Function4/1(e_out) -> Err/1
  MATLAB Function2/1(Oy) -> MATLAB Function4/1(Oy)
  Subtract2/1 -> MATLAB Function4/2(e_in)
  MATLAB Function2/2(Ox) -> Subtract2/1
  Act/1 -> MATLAB Function3/1(z)
  Ref/1 -> MATLAB Function2/1(z)
  MATLAB Function3/1(Ox) -> Subtract2/2

== system combined_experiment/Phase #5: Hold Home/Change RED Behavior/Custom Discrete PD (Attitude) ==
  ez : Inport
  Sum3 : Sum
  kd_tr : Gain  Gain=Kd_tr
  kp_tr : Gain  Gain=Kp_tr
  "x_dot -> x1" : Subsystem
  Tz : Outport  VectorParamsAs1DForOutWhenUnconnected=off
  wires:
  kd_tr/1 -> Sum3/1
  Sum3/1 -> Tz/1
  kp_tr/1 -> Sum3/2
  "x_dot -> x1"/1(dy(t)/dt) -> kd_tr/1
  ez/1 -> "x_dot -> x1"/1(y(t)), kp_tr/1

== system combined_experiment/Phase #5: Hold Home/Change RED Behavior/Custom Discrete PD (X-Position) ==
  ex : Inport
  Sum3 : Sum
  kd_xr : Gain  Gain=Kd_xr
  kp_xr : Gain  Gain=Kp_xr
  "x_dot -> x1" : Subsystem
  Fx : Outport  VectorParamsAs1DForOutWhenUnconnected=off
  wires:
  kd_xr/1 -> Sum3/1
  ex/1 -> "x_dot -> x1"/1(y(t)), kp_xr/1
  kp_xr/1 -> Sum3/2
  "x_dot -> x1"/1(dy(t)/dt) -> kd_xr/1
  Sum3/1 -> Fx/1

== system combined_experiment/Phase #5: Hold Home/Change RED Behavior/Custom Discrete PD (Y-Position) ==
  ey : Inport
  Sum3 : Sum
  kd_yr : Gain  Gain=Kd_yr
  kp_yr : Gain  Gain=Kp_yr
  "x_dot -> x1" : Subsystem
  Fy : Outport  VectorParamsAs1DForOutWhenUnconnected=off
  wires:
  kd_yr/1 -> Sum3/1
  Sum3/1 -> Fy/1
  kp_yr/1 -> Sum3/2
  "x_dot -> x1"/1(dy(t)/dt) -> kd_yr/1
  ey/1 -> "x_dot -> x1"/1(y(t)), kp_yr/1

== system combined_experiment/Phase #5: Hold Home/Change RED Behavior/Hough Control ==
  Ref : Inport
  Act : Inport  Port=2
  MATLAB Function2 : MATLAB Function  TreatAsAtomicUnit=on
  MATLAB Function3 : MATLAB Function  TreatAsAtomicUnit=on
  MATLAB Function4 : MATLAB Function  TreatAsAtomicUnit=on
  Subtract2 : Sum  Inputs=+-
  Err : Outport  VectorParamsAs1DForOutWhenUnconnected=off
  wires:
  MATLAB Function4/1(e_out) -> Err/1
  MATLAB Function2/1(Oy) -> MATLAB Function4/1(Oy)
  Subtract2/1 -> MATLAB Function4/2(e_in)
  MATLAB Function2/2(Ox) -> Subtract2/1
  Act/1 -> MATLAB Function3/1(z)
  Ref/1 -> MATLAB Function2/1(z)
  MATLAB Function3/1(Ox) -> Subtract2/2

== system combined_experiment/Simulate Plant Dynamics/x_dot -> x1/Hold this value ==
  In1 : Inport
  Action Port : ActionPort  ActionPortLabel=if(u1 ~= 0)
  Out1 : Outport  VectorParamsAs1DForOutWhenUnconnected=off
  wires:
  In1/1 -> Out1/1

== system combined_experiment/Simulate Plant Dynamics/x_dot -> x10/Hold this value ==
  In1 : Inport
  Action Port : ActionPort  ActionPortLabel=if(u1 ~= 0)
  Out1 : Outport  VectorParamsAs1DForOutWhenUnconnected=off
  wires:
  In1/1 -> Out1/1

== system combined_experiment/Simulate Plant Dynamics/x_dot -> x11/Hold this value ==
  In1 : Inport
  Action Port : ActionPort  ActionPortLabel=if(u1 ~= 0)
  Out1 : Outport  VectorParamsAs1DForOutWhenUnconnected=off
  wires:
  In1/1 -> Out1/1

== system combined_experiment/Simulate Plant Dynamics/x_dot -> x12/Hold this value ==
  In1 : Inport
  Action Port : ActionPort  ActionPortLabel=if(u1 ~= 0)
  Out1 : Outport  VectorParamsAs1DForOutWhenUnconnected=off
  wires:
  In1/1 -> Out1/1

== system combined_experiment/Simulate Plant Dynamics/x_dot -> x13/Hold this value ==
  In1 : Inport
  Action Port : ActionPort  ActionPortLabel=if(u1 ~= 0)
  Out1 : Outport  VectorParamsAs1DForOutWhenUnconnected=off
  wires:
  In1/1 -> Out1/1

== system combined_experiment/Simulate Plant Dynamics/x_dot -> x14/Hold this value ==
  In1 : Inport
  Action Port : ActionPort  ActionPortLabel=if(u1 ~= 0)
  Out1 : Outport  VectorParamsAs1DForOutWhenUnconnected=off
  wires:
  In1/1 -> Out1/1

== system combined_experiment/Simulate Plant Dynamics/x_dot -> x16/Hold this value ==
  In1 : Inport
  Action Port : ActionPort  ActionPortLabel=if(u1 ~= 0)
  Out1 : Outport  VectorParamsAs1DForOutWhenUnconnected=off
  wires:
  In1/1 -> Out1/1

== system combined_experiment/Simulate Plant Dynamics/x_dot -> x17/Hold this value ==
  In1 : Inport
  Action Port : ActionPort  ActionPortLabel=if(u1 ~= 0)
  Out1 : Outport  VectorParamsAs1DForOutWhenUnconnected=off
  wires:
  In1/1 -> Out1/1

== system combined_experiment/Simulate Plant Dynamics/x_dot -> x2/Hold this value ==
  In1 : Inport
  Action Port : ActionPort  ActionPortLabel=if(u1 ~= 0)
  Out1 : Outport  VectorParamsAs1DForOutWhenUnconnected=off
  wires:
  In1/1 -> Out1/1

== system combined_experiment/Simulate Plant Dynamics/x_dot -> x3/Hold this value ==
  In1 : Inport
  Action Port : ActionPort  ActionPortLabel=if(u1 ~= 0)
  Out1 : Outport  VectorParamsAs1DForOutWhenUnconnected=off
  wires:
  In1/1 -> Out1/1

== system combined_experiment/Simulate Plant Dynamics/x_dot -> x4/Hold this value ==
  In1 : Inport
  Action Port : ActionPort  ActionPortLabel=if(u1 ~= 0)
  Out1 : Outport  VectorParamsAs1DForOutWhenUnconnected=off
  wires:
  In1/1 -> Out1/1

== system combined_experiment/Simulate Plant Dynamics/x_dot -> x5/Hold this value ==
  In1 : Inport
  Action Port : ActionPort  ActionPortLabel=if(u1 ~= 0)
  Out1 : Outport  VectorParamsAs1DForOutWhenUnconnected=off
  wires:
  In1/1 -> Out1/1

== system combined_experiment/Simulate Plant Dynamics/x_dot -> x6/Hold this value ==
  In1 : Inport
  Action Port : ActionPort  ActionPortLabel=if(u1 ~= 0)
  Out1 : Outport  VectorParamsAs1DForOutWhenUnconnected=off
  wires:
  In1/1 -> Out1/1

== system combined_experiment/Simulate Plant Dynamics/x_dot -> x7/Hold this value ==
  In1 : Inport
  Action Port : ActionPort  ActionPortLabel=if(u1 ~= 0)
  Out1 : Outport  VectorParamsAs1DForOutWhenUnconnected=off
  wires:
  In1/1 -> Out1/1

== system combined_experiment/Simulate Plant Dynamics/x_dot -> x8/Hold this value ==
  In1 : Inport
  Action Port : ActionPort  ActionPortLabel=if(u1 ~= 0)
  Out1 : Outport  VectorParamsAs1DForOutWhenUnconnected=off
  wires:
  In1/1 -> Out1/1

== system combined_experiment/Simulate Plant Dynamics/x_dot -> x9/Hold this value ==
  In1 : Inport
  Action Port : ActionPort  ActionPortLabel=if(u1 ~= 0)
  Out1 : Outport  VectorParamsAs1DForOutWhenUnconnected=off
  wires:
  In1/1 -> Out1/1

== system combined_experiment/From Force//Torque to PWM Signal/Change BLACK Behavior/Calculate Thruster ON//OFF/Rotate Forces to Inertial ==
  "F_b " : Inport
  Rz : Inport  Port=2
  Create Rotation Matrix : MATLAB Function  TreatAsAtomicUnit=on
  Rotate F_b to F_I : Product  Multiplication=Matrix(*)
  F_I : Outport  VectorParamsAs1DForOutWhenUnconnected=off
  wires:
  "F_b "/1 -> Rotate F_b to F_I/2
  Rotate F_b to F_I/1 -> F_I/1
  Create Rotation Matrix/1(C_Ib) -> Rotate F_b to F_I/1
  Rz/1 -> Create Rotation Matrix/1(Rz)

== system combined_experiment/From Force//Torque to PWM Signal/Change BLACK Behavior/Calculate Thruster ON//OFF/pseudo-inverse ==
  H : Inport
  Product : Product  Multiplication=Matrix(*)
  Product1 : Product  Inputs=/  Multiplication=Matrix(*)
  Product2 : Product  Multiplication=Matrix(*)
  transpose : PermuteDimensions
  invH : Outport  VectorParamsAs1DForOutWhenUnconnected=off
  wires:
  Product2/1 -> invH/1
  transpose/1 -> Product/2, Product2/1
  Product/1 -> Product1/1
  H/1 -> Product/1, transpose/1
  Product1/1 -> Product2/2

== system combined_experiment/From Force//Torque to PWM Signal/Change BLUE Behavior/Calculate Thruster ON//OFF/Rotate Forces to Inertial ==
  "F_b " : Inport
  Rz : Inport  Port=2
  Create Rotation Matrix : MATLAB Function  TreatAsAtomicUnit=on
  Rotate F_b to F_I : Product  Multiplication=Matrix(*)
  F_I : Outport  VectorParamsAs1DForOutWhenUnconnected=off
  wires:
  "F_b "/1 -> Rotate F_b to F_I/2
  Rotate F_b to F_I/1 -> F_I/1
  Create Rotation Matrix/1(C_Ib) -> Rotate F_b to F_I/1
  Rz/1 -> Create Rotation Matrix/1(Rz)

== system combined_experiment/From Force//Torque to PWM Signal/Change BLUE Behavior/Calculate Thruster ON//OFF/pseudo-inverse ==
  H : Inport
  Product : Product  Multiplication=Matrix(*)
  Product1 : Product  Inputs=/  Multiplication=Matrix(*)
  Product2 : Product  Multiplication=Matrix(*)
  transpose : PermuteDimensions
  invH : Outport  VectorParamsAs1DForOutWhenUnconnected=off
  wires:
  Product2/1 -> invH/1
  transpose/1 -> Product/2, Product2/1
  Product/1 -> Product1/1
  H/1 -> Product/1, transpose/1
  Product1/1 -> Product2/2

== system combined_experiment/From Force//Torque to PWM Signal/Change RED Behavior/Calculate Thruster ON//OFF/Rotate Forces to Inertial ==
  "F_b " : Inport
  Rz : Inport  Port=2
  Create Rotation Matrix : MATLAB Function  TreatAsAtomicUnit=on
  Rotate F_b to F_I : Product  Multiplication=Matrix(*)
  F_I : Outport  VectorParamsAs1DForOutWhenUnconnected=off
  wires:
  "F_b "/1 -> Rotate F_b to F_I/2
  Rotate F_b to F_I/1 -> F_I/1
  Create Rotation Matrix/1(C_Ib) -> Rotate F_b to F_I/1
  Rz/1 -> Create Rotation Matrix/1(Rz)

== system combined_experiment/From Force//Torque to PWM Signal/Change RED Behavior/Calculate Thruster ON//OFF/pseudo-inverse ==
  H : Inport
  Product : Product  Multiplication=Matrix(*)
  Product1 : Product  Inputs=/  Multiplication=Matrix(*)
  Product2 : Product  Multiplication=Matrix(*)
  transpose : PermuteDimensions
  invH : Outport  VectorParamsAs1DForOutWhenUnconnected=off
  wires:
  Product2/1 -> invH/1
  transpose/1 -> Product/2, Product2/1
  Product/1 -> Product1/1
  H/1 -> Product/1, transpose/1
  Product1/1 -> Product2/2

== system combined_experiment/From Force//Torque to PWM Signal/Change RED Behavior/Calculate Thruster ON//OFF/pseudo-inverse1 ==
  H : Inport
  Product : Product  Multiplication=Matrix(*)
  Product1 : Product  Inputs=/  Multiplication=Matrix(*)
  Product2 : Product  Multiplication=Matrix(*)
  transpose : PermuteDimensions
  invH : Outport  VectorParamsAs1DForOutWhenUnconnected=off
  wires:
  Product2/1 -> invH/1
  transpose/1 -> Product/2, Product2/1
  Product/1 -> Product1/1
  H/1 -> Product/1, transpose/1
  Product1/1 -> Product2/2

== system combined_experiment/From Torque, Command RW/Change RED Behavior/Wheel RPM to PWM/Convert Wheel Rate to Motor Rate ==
  Wheel RPM : Inport
  Divide : Product  Inputs=**
  Gearbox Ratio : Constant  Value=3375/64
  Motor RPM : Outport  VectorParamsAs1DForOutWhenUnconnected=off
  wires:
  Gearbox Ratio/1 -> Divide/2
  Divide/1 -> Motor RPM/1
  Wheel RPM/1 -> Divide/1

== system combined_experiment/From Torque, Command RW/Change RED Behavior/Wheel RPM to PWM/Delay Bank ==
  Status : Inport
  Delay1 : Delay  DelayLength=1  InitialCondition=0
  Delay2 : Delay  InitialCondition=0
  Delay3 : Delay  DelayLength=4  InitialCondition=0
  Delay4 : Delay  DelayLength=5  InitialCondition=0
  Delay5 : Delay  DelayLength=3  InitialCondition=0
  Mostly zeros? : MinMax  Inputs=6
  StatusVector : Outport  VectorParamsAs1DForOutWhenUnconnected=off
  wires:
  Delay3/1 -> Mostly zeros?/5
  Status/1 -> Delay4/1, Delay3/1, Delay5/1, Delay2/1, Delay1/1, Mostly zeros?/1
  Delay2/1 -> Mostly zeros?/3
  Delay4/1 -> Mostly zeros?/6
  Delay5/1 -> Mostly zeros?/4
  Mostly zeros?/1 -> StatusVector/1
  Delay1/1 -> Mostly zeros?/2

== system combined_experiment/From Torque, Command RW/Change RED Behavior/Wheel RPM to PWM/Obtain RW Status ==
  GPIO Read1 : embdlinuxlib/GPIO Read  board=Pi 3 Model B  gpio=24  internalResistor=Off  sampleTime=0.1  direction=Input  blockPlatform=Raspberry Pi
      settings: SourceProductBaseCode=SC_BEAGLEBONE_BLUE,RASPPI
  RW_Status : Outport  VectorParamsAs1DForOutWhenUnconnected=off
  wires:
  GPIO Read1/1 -> RW_Status/1

== system combined_experiment/From Torque, Command RW/Change RED Behavior/Wheel RPM to PWM/Send Direction to Motor Controller ==
  WheelDir : Inport
  GPIO Write : embdlinuxlib/GPIO Write  board=Pi 3 Model B  gpio=21  direction=Output  blockPlatform=Raspberry Pi
      settings: SourceProductBaseCode=SC_BEAGLEBONE_BLUE,RASPPI
  wires:
  WheelDir/1 -> GPIO Write/1

== system combined_experiment/From Torque, Command RW/Change RED Behavior/Wheel RPM to PWM/Send PWM to Motor Controller ==
  MotorPWM : Inport
  PWM1 : raspberrypiBasiclib/PWM  board=Pi 3 Model B  Pin_=18  Frequency=10  blockPlatform=Raspberry Pi
      settings: SourceProductBaseCode=RASPPI
  wires:
  MotorPWM/1 -> PWM1/1

== system combined_experiment/From Torque, Command RW/Change RED Behavior/Wheel RPM to PWM/Turn on Motor ==
  EnableSig : Inport
  GPIO Write1 : embdlinuxlib/GPIO Write  board=Pi 3 Model B  gpio=25  direction=Output  blockPlatform=Raspberry Pi
      settings: SourceProductBaseCode=SC_BEAGLEBONE_BLUE,RASPPI
  wires:
  EnableSig/1 -> GPIO Write1/1

== system combined_experiment/Grab PhaseSpace Data via UDP/Use Hardware to Obtain States/Using RED+BLACK, or RED+BLACK+ARM/Is this a simulation? ==
  Constant : Constant  Value=simMode  SampleTime=-1
  isSim : Outport  VectorParamsAs1DForOutWhenUnconnected=off
  wires:
  Constant/1 -> isSim/1
